simulink model "compensacion_digital"  (R2014b)
settings: Solver=ode45  StartTime=0.0  StopTime=4  RelTol=1e-3
settings Model: Creator=Javi  LastModifiedBy=Javi

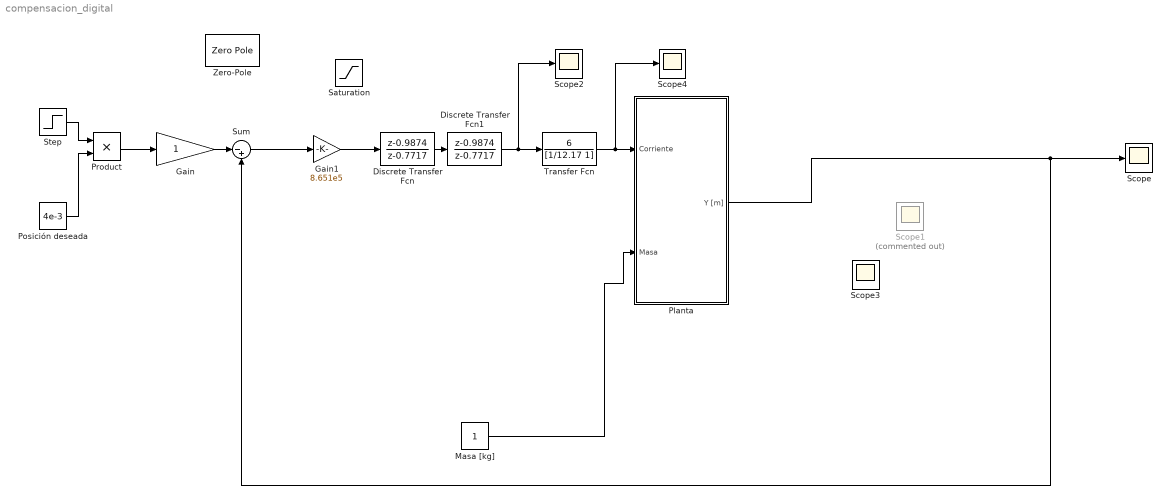
== system compensacion_digital ==
  Discrete Transfer Fcn : DiscreteTransferFcn  Numerator=[1 -0.9874]  Denominator=[1 -0.7717]  SampleTime=1/3.5e3
  Discrete Transfer Fcn1 : DiscreteTransferFcn  Numerator=[1 -0.9874]  Denominator=[1 -0.7717]
  Gain : Gain
  Gain1 : Gain  Gain=8.651e5
  "Masa [kg] " : Constant
  "Planta " : Subsystem
  Posición deseada : Constant  Value=4e-3
  Product : Product
  Saturation : Saturate  UpperLimit=5  LowerLimit=-inf
  Scope{,2..4} (4 alike) : Scope
      Scope settings: TimeRange=4  YMin=0  YMax=0.014
      Scope2 settings: TimeRange=0.1028681317068158  YMin=-4000  YMax=5000  SaveName=ScopeData2
      Scope3 settings: TimeRange=4  YMin=-400000  YMax=600000  SaveName=ScopeData3
      Scope4 settings: TimeRange=0.005185185185185187  YMin=-3500000  YMax=500000  SaveName=ScopeData4
  Scope1 : Scope  Commented=on
  Step : Step  Time=0.01  SampleTime=0
  Sum : Sum  Inputs=|-+
  Transfer Fcn : TransferFcn  Numerator=[6]  Denominator=[1/12.17 1]
  Zero-Pole : ZeroPole  Zeros=[-221.7 -221.7]  Poles=[-4511 -4511]  Gain=8.28e5
  wires:
  "Masa [kg] "/1 -> "Planta "/2("Masa ")
  ? -> Scope1/1
  Gain/1 -> Sum/1
  "Planta "/1(Y [m]) -> Sum/2, Scope/1
  Transfer Fcn/1 -> "Planta "/1(Corriente), Scope4/1
  ? -> Scope3/1
  Discrete Transfer Fcn1/1 -> Scope2/1, Transfer Fcn/1
  Step/1 -> Product/1
  Posición deseada/1 -> Product/2
  Product/1 -> Gain/1
  Gain1/1 -> Discrete Transfer Fcn/1
  Sum/1 -> Gain1/1
  Discrete Transfer Fcn/1 -> Discrete Transfer Fcn1/1

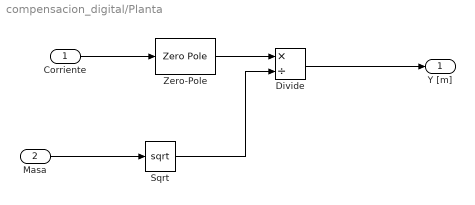
== system compensacion_digital/Planta  ==
  Corriente : Inport
  "Masa " : Inport  Port=2
  Divide : Product  Inputs=*/
  Sqrt : Sqrt  SaturateOnIntegerOverflow=on
  Zero-Pole : ZeroPole  Zeros=[]  Poles=[70 -70]  Gain=-6.58
  Y [m] : Outport
  wires:
  Divide/1 -> Y [m]/1
  Corriente/1 -> Zero-Pole/1
  Zero-Pole/1 -> Divide/1
  "Masa "/1 -> Sqrt/1
  Sqrt/1 -> Divide/2
